simulink model "EPD629_WilliamsJ_AS05_simulink"  (R2021b)
settings: Solver=VariableStepAuto  StartTime=0.0  StopTime=1.5  RelTol=1e-3
values from neighbouring files (symbols this model uses):
  ArmatureVoltage = 10    [EPD629_WilliamsJ_AS05.m]
  b = 0.001    [EPD629_WilliamsJ_AS05.m]
  J = 50e-6    (= 5e-05)    [EPD629_WilliamsJ_AS05.m]
  K = 0.1    [EPD629_WilliamsJ_AS05.m]
  Kb = Kt    (= 0.063)    [EPD629_WilliamsJ_AS05.m]
  Kint = 1.5    [EPD629_WilliamsJ_AS05.m]
  Kprop = 3    [EPD629_WilliamsJ_AS05.m]
  Kt = 0.063    [EPD629_WilliamsJ_AS05.m]
  L = 1e-3    (= 0.001)    [EPD629_WilliamsJ_AS05.m]
  R = 0.35    [EPD629_WilliamsJ_AS05.m]
settings Model: Creator=jwilli42  LastModifiedBy=justin

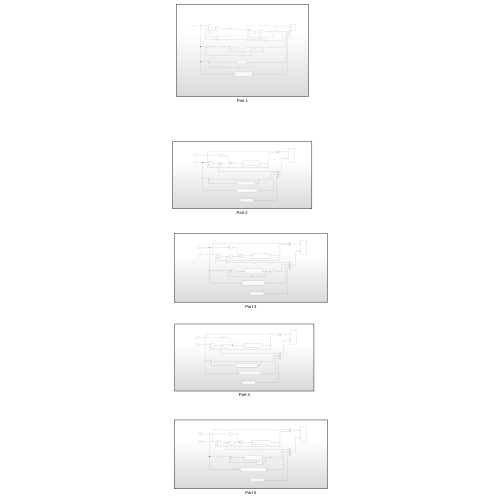
[thumbnail: Simulink's stored preview of the top-level diagram]
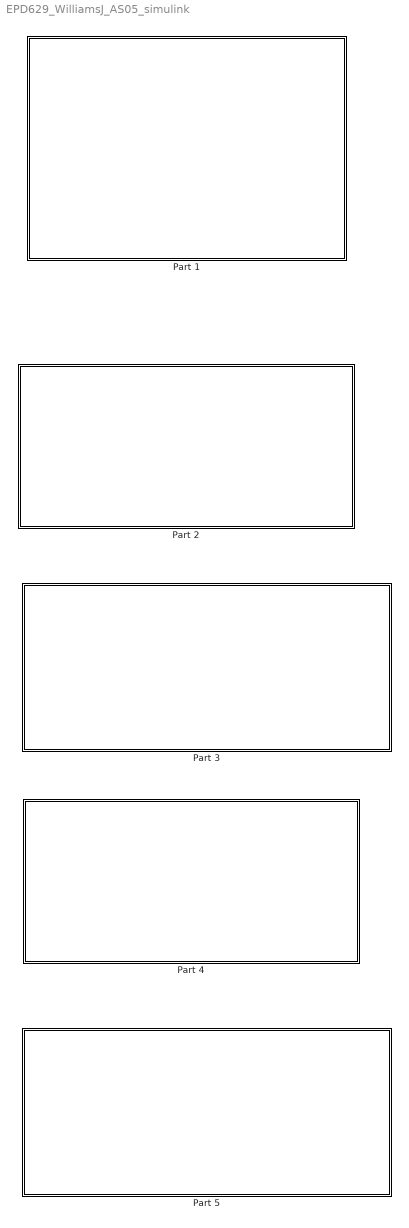
== system EPD629_WilliamsJ_AS05_simulink ==
  Part 1 : Subsystem
  Part 2 : Subsystem
  Part 3 : Subsystem
  Part 4 : Subsystem
  Part 5 : Subsystem

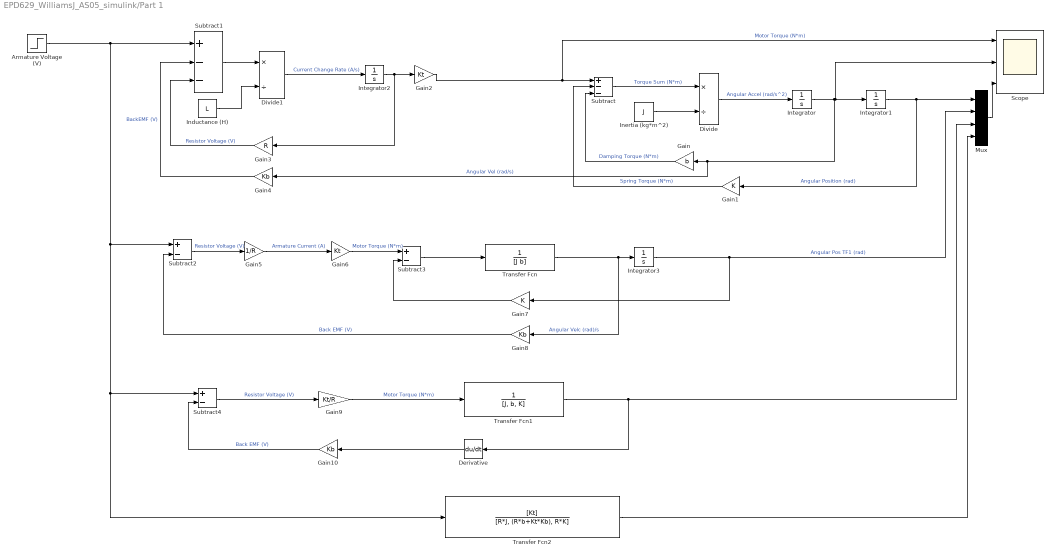
== system EPD629_WilliamsJ_AS05_simulink/Part 1 ==
  Armature Voltage (V) : Step  Time=0  After=ArmatureVoltage  SampleTime=0
  Derivative : Derivative
  Divide : Product  Inputs=*/
  Divide1 : Product  Inputs=*/
  Gain : Gain  Gain=b
  Gain1 : Gain  Gain=K
  Gain10 : Gain  Gain=Kb
  Gain2 : Gain  Gain=Kt
  Gain3 : Gain  Gain=R
  Gain4 : Gain  Gain=Kb
  Gain5 : Gain  Gain=1/R
  Gain6 : Gain  Gain=Kt
  Gain7 : Gain  Gain=K
  Gain8 : Gain  Gain=Kb
  Gain9 : Gain  Gain=Kt/R
  Inductance (H) : Constant  Value=L
  Inertia (kg*m^2) : Constant  Value=J
  Integrator{,1..3} (4 alike) : Integrator
  Mux : Mux
  Scope : Scope  NumInputPorts=3
  Subtract : Sum  Inputs=+--
  Subtract1 : Sum  Inputs=+--
  Subtract2 : Sum  Inputs=+-
  Subtract3 : Sum  Inputs=+-
  Subtract4 : Sum  Inputs=+-
  Transfer Fcn : TransferFcn  Denominator=[J b]
  Transfer Fcn1 : TransferFcn  Denominator=[J, b, K]
  Transfer Fcn2 : TransferFcn  Numerator=[Kt]  Denominator=[R*J, (R*b+Kt*Kb), R*K]
  wires:
  Divide/1 -> Integrator/1  "Angular Accel (rad/s^2)"
  Gain6/1 -> Subtract3/1  "Motor Torque (N*m)"
  Integrator3/1 -> Gain7/1, Mux/2  "Angular Pos TF1 (rad)"
  Gain2/1 -> Scope/1, Subtract/1  "Motor Torque (N*m)"
  Subtract2/1 -> Gain5/1  "Resistor Voltage (V)"
  Gain1/1 -> Subtract/2  "Spring Torque (N*m)"
  Transfer Fcn1/1 -> Derivative/1, Mux/3
  Gain8/1 -> Subtract2/2  "Back EMF (V)"
  Gain7/1 -> Subtract3/2
  Subtract/1 -> Divide/1  "Torque Sum (N*m)"
  Transfer Fcn/1 -> Gain8/1, Integrator3/1  "Angular Velc (rad)/s"
  Inertia (kg*m^2)/1 -> Divide/2
  Divide1/1 -> Integrator2/1  "Current Change Rate (A/s)"
  Armature Voltage (V)/1 -> Transfer Fcn2/1, Subtract4/1, Subtract2/1, Subtract1/1
  Subtract4/1 -> Gain9/1  "Resistor Voltage (V)"
  Integrator1/1 -> Gain1/1, Mux/1  "Angular Position (rad)"
  Transfer Fcn2/1 -> Mux/4
  Gain5/1 -> Gain6/1  "Armature Current (A)"
  Integrator2/1 -> Gain3/1, Gain2/1
  Gain3/1 -> Subtract1/3  "Resistor Voltage (V)"
  Inductance (H)/1 -> Divide1/2
  Gain4/1 -> Subtract1/2  "BackEMF (V)"
  Subtract3/1 -> Transfer Fcn/1
  Gain9/1 -> Transfer Fcn1/1  "Motor Torque (N*m)"
  Subtract1/1 -> Divide1/1
  Mux/1 -> Scope/3
  Integrator/1 -> Scope/2, Integrator1/1, Gain/1, Gain4/1  "Angular Vel (rad/s)"
  Gain/1 -> Subtract/3  "Damping Torque (N*m)"
  Derivative/1 -> Gain10/1
  Gain10/1 -> Subtract4/2  "Back EMF (V)"

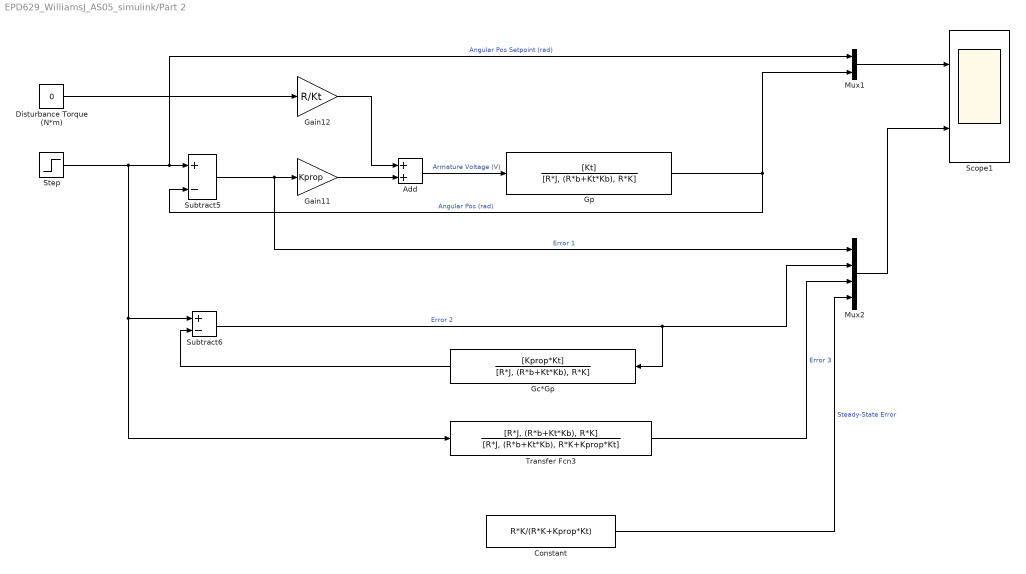
== system EPD629_WilliamsJ_AS05_simulink/Part 2 ==
  Add : Sum
  Constant : Constant  Value=R*K/(R*K+Kprop*Kt)
  Disturbance Torque (N*m) : Constant  Value=0
  Gain11 : Gain  Gain=Kprop
  Gain12 : Gain  Gain=R/Kt
  Gc*Gp : TransferFcn  Numerator=[Kprop*Kt]  Denominator=[R*J, (R*b+Kt*Kb), R*K]
  Gp : TransferFcn  Numerator=[Kt]  Denominator=[R*J, (R*b+Kt*Kb), R*K]
  Mux1 : Mux  Inputs=2
  Mux2 : Mux
  Scope1 : Scope  NumInputPorts=2
  Step : Step  Time=0  SampleTime=0
  Subtract5 : Sum  Inputs=+-
  Subtract6 : Sum  Inputs=+-
  Transfer Fcn3 : TransferFcn  Numerator=[R*J, (R*b+Kt*Kb), R*K]  Denominator=[R*J, (R*b+Kt*Kb), R*K+Kprop*Kt]
  wires:
  Add/1 -> Gp/1  "Armature Voltage (V)"
  Mux1/1 -> Scope1/1
  Constant/1 -> Mux2/4  "Steady-State Error"
  Mux2/1 -> Scope1/2
  Gain11/1 -> Add/2
  Transfer Fcn3/1 -> Mux2/3  "Error 3"
  Gain12/1 -> Add/1
  Disturbance Torque (N*m)/1 -> Gain12/1
  Step/1 -> Transfer Fcn3/1, Subtract6/1, Subtract5/1, Mux1/1  "Angular Pos Setpoint (rad)"
  Gp/1 -> Subtract5/2, Mux1/2  "Angular Pos (rad)"
  Gc*Gp/1 -> Subtract6/2
  Subtract6/1 -> Gc*Gp/1, Mux2/2  "Error 2"
  Subtract5/1 -> Mux2/1, Gain11/1  "Error 1"

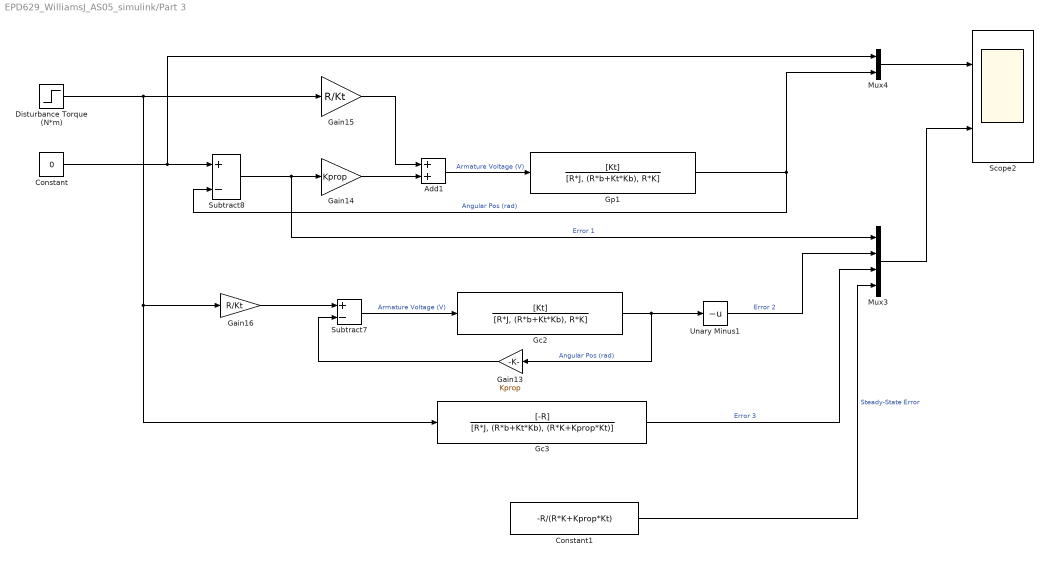
== system EPD629_WilliamsJ_AS05_simulink/Part 3 ==
  Add1 : Sum
  Constant : Constant  Value=0
  Constant1 : Constant  Value=-R/(R*K+Kprop*Kt)
  Disturbance Torque (N*m) : Step  Time=0  SampleTime=0
  Gain13 : Gain  Gain=Kprop
  Gain14 : Gain  Gain=Kprop
  Gain15 : Gain  Gain=R/Kt
  Gain16 : Gain  Gain=R/Kt
  Gc2 : TransferFcn  Numerator=[Kt]  Denominator=[R*J, (R*b+Kt*Kb), R*K]
  Gc3 : TransferFcn  Numerator=[-R]  Denominator=[R*J, (R*b+Kt*Kb), (R*K+Kprop*Kt)]
  Gp1 : TransferFcn  Numerator=[Kt]  Denominator=[R*J, (R*b+Kt*Kb), R*K]
  Mux3 : Mux
  Mux4 : Mux  Inputs=2
  Scope2 : Scope  NumInputPorts=2
  Subtract7 : Sum  Inputs=+-
  Subtract8 : Sum  Inputs=+-
  Unary Minus1 : UnaryMinus
  wires:
  Gain14/1 -> Add1/2
  Unary Minus1/1 -> Mux3/2  "Error 2"
  Constant1/1 -> Mux3/4  "Steady-State Error"
  Gc3/1 -> Mux3/3  "Error 3"
  Subtract8/1 -> Gain14/1, Mux3/1  "Error 1"
  Gc2/1 -> Gain13/1, Unary Minus1/1  "Angular Pos (rad)"
  Gain16/1 -> Subtract7/1
  Gp1/1 -> Mux4/2, Subtract8/2  "Angular Pos (rad)"
  Gain15/1 -> Add1/1
  Mux3/1 -> Scope2/2
  Disturbance Torque (N*m)/1 -> Gain16/1, Gc3/1, Gain15/1
  Gain13/1 -> Subtract7/2
  Subtract7/1 -> Gc2/1  "Armature Voltage (V)"
  Mux4/1 -> Scope2/1
  Add1/1 -> Gp1/1  "Armature Voltage (V)"
  Constant/1 -> Subtract8/1, Mux4/1

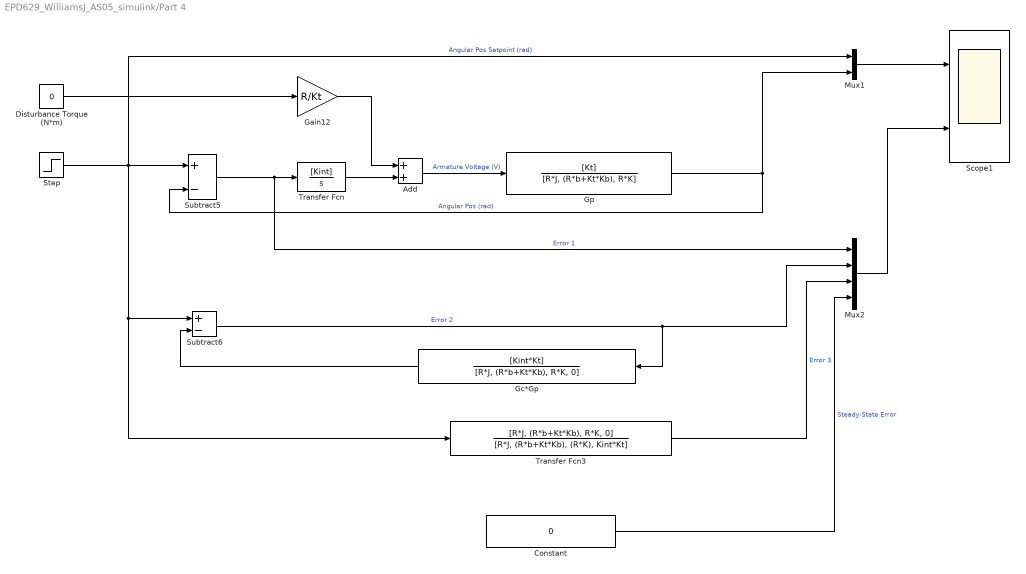
== system EPD629_WilliamsJ_AS05_simulink/Part 4 ==
  Add : Sum
  Constant : Constant  Value=0
  Disturbance Torque (N*m) : Constant  Value=0
  Gain12 : Gain  Gain=R/Kt
  Gc*Gp : TransferFcn  Numerator=[Kint*Kt]  Denominator=[R*J, (R*b+Kt*Kb), R*K, 0]
  Gp : TransferFcn  Numerator=[Kt]  Denominator=[R*J, (R*b+Kt*Kb), R*K]
  Mux1 : Mux  Inputs=2
  Mux2 : Mux
  Scope1 : Scope  NumInputPorts=2
  Step : Step  Time=0  SampleTime=0
  Subtract5 : Sum  Inputs=+-
  Subtract6 : Sum  Inputs=+-
  Transfer Fcn : TransferFcn  Numerator=[Kint]  Denominator=[1 0]
  Transfer Fcn3 : TransferFcn  Numerator=[R*J, (R*b+Kt*Kb), R*K, 0]  Denominator=[R*J, (R*b+Kt*Kb), (R*K), Kint*Kt]
  wires:
  Subtract5/1 -> Mux2/1, Transfer Fcn/1  "Error 1"
  Subtract6/1 -> Mux2/2, Gc*Gp/1  "Error 2"
  Gp/1 -> Mux1/2, Subtract5/2  "Angular Pos (rad)"
  Step/1 -> Subtract5/1, Mux1/1, Subtract6/1, Transfer Fcn3/1  "Angular Pos Setpoint (rad)"
  Disturbance Torque (N*m)/1 -> Gain12/1
  Gain12/1 -> Add/1
  Transfer Fcn3/1 -> Mux2/3  "Error 3"
  Transfer Fcn/1 -> Add/2
  Mux2/1 -> Scope1/2
  Constant/1 -> Mux2/4  "Steady-State Error"
  Mux1/1 -> Scope1/1
  Add/1 -> Gp/1  "Armature Voltage (V)"
  Gc*Gp/1 -> Subtract6/2

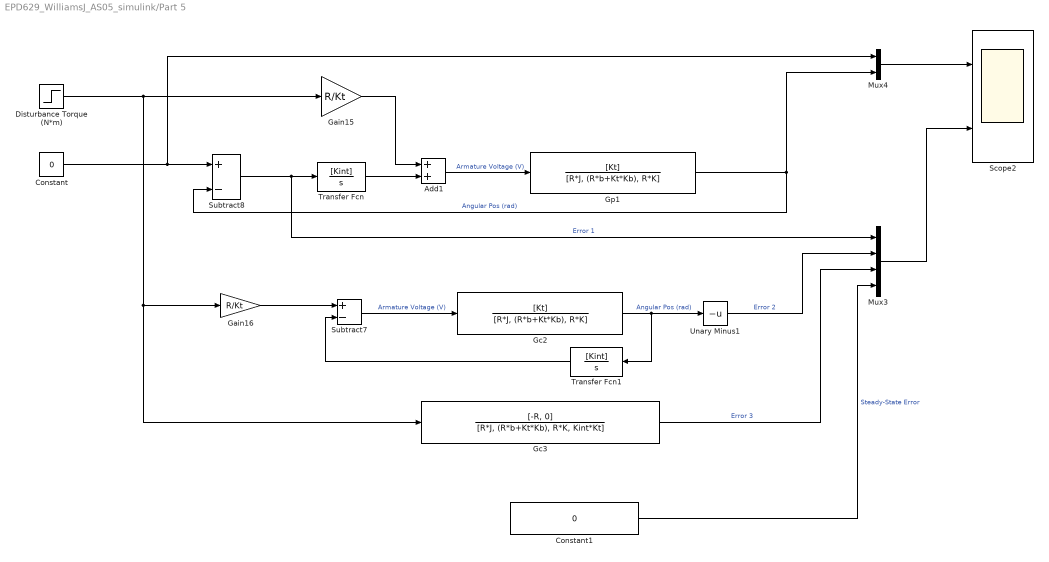
== system EPD629_WilliamsJ_AS05_simulink/Part 5 ==
  Add1 : Sum
  Constant : Constant  Value=0
  Constant1 : Constant  Value=0
  Disturbance Torque (N*m) : Step  Time=0  SampleTime=0
  Gain15 : Gain  Gain=R/Kt
  Gain16 : Gain  Gain=R/Kt
  Gc2 : TransferFcn  Numerator=[Kt]  Denominator=[R*J, (R*b+Kt*Kb), R*K]
  Gc3 : TransferFcn  Numerator=[-R, 0]  Denominator=[R*J, (R*b+Kt*Kb), R*K, Kint*Kt]
  Gp1 : TransferFcn  Numerator=[Kt]  Denominator=[R*J, (R*b+Kt*Kb), R*K]
  Mux3 : Mux
  Mux4 : Mux  Inputs=2
  Scope2 : Scope  NumInputPorts=2
  Subtract7 : Sum  Inputs=+-
  Subtract8 : Sum  Inputs=+-
  Transfer Fcn : TransferFcn  Numerator=[Kint]  Denominator=[1 0]
  Transfer Fcn1 : TransferFcn  Numerator=[Kint]  Denominator=[1 0]
  Unary Minus1 : UnaryMinus
  wires:
  Constant/1 -> Mux4/1, Subtract8/1
  Add1/1 -> Gp1/1  "Armature Voltage (V)"
  Mux4/1 -> Scope2/1
  Subtract7/1 -> Gc2/1  "Armature Voltage (V)"
  Transfer Fcn1/1 -> Subtract7/2
  Disturbance Torque (N*m)/1 -> Gain15/1, Gc3/1, Gain16/1
  Mux3/1 -> Scope2/2
  Gain15/1 -> Add1/1
  Gp1/1 -> Subtract8/2, Mux4/2  "Angular Pos (rad)"
  Gain16/1 -> Subtract7/1
  Gc2/1 -> Transfer Fcn1/1, Unary Minus1/1  "Angular Pos (rad)"
  Subtract8/1 -> Transfer Fcn/1, Mux3/1  "Error 1"
  Gc3/1 -> Mux3/3  "Error 3"
  Constant1/1 -> Mux3/4  "Steady-State Error"
  Unary Minus1/1 -> Mux3/2  "Error 2"
  Transfer Fcn/1 -> Add1/2
